simulink model "MVC3"  (R2019b)
settings: Solver=VariableStepAuto  StartTime=0.0  StopTime=SimulationTime  RelTol=1e-3
values from neighbouring files (symbols this model uses):
  disturbanceStrength = 0.001    [Obliczenia.m]
  SampleTime = 1    [Obliczenia.m]
libraries: simulink x5
settings Model: Creator=pleka  LastModifiedBy=pleka

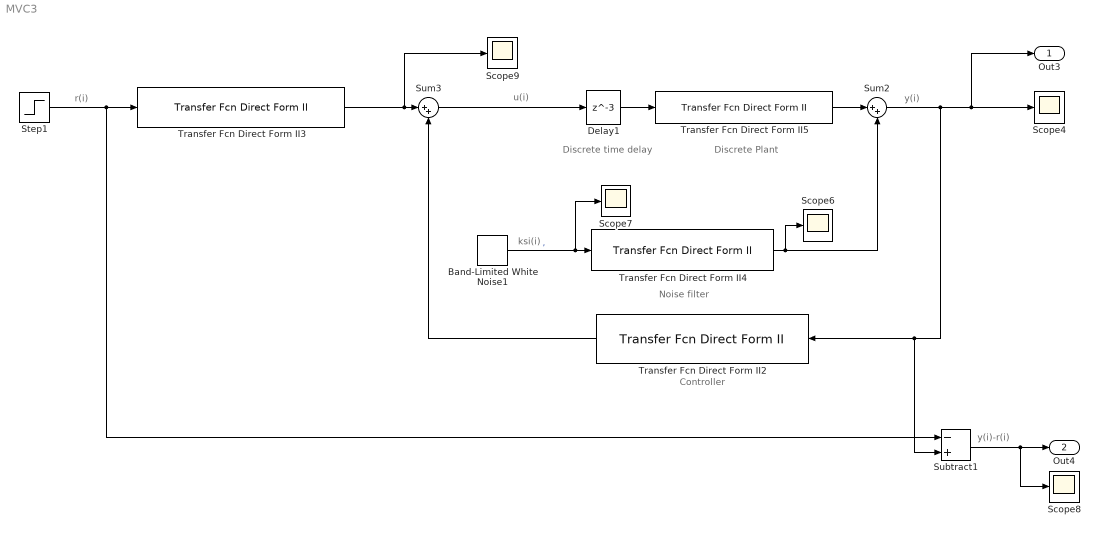
== system MVC3 ==
  note: Discrete Plant
  note: u(i)
  note: Discrete time delay
  note: Noise filter
  note: Controller
  note: r(i)
  note: y(i)-r(i)
  note: y(i)
  note: ksi(i)
  Band-Limited White Noise1 : simulink/Sources/Band-Limited White Noise  Cov=[disturbanceStrength]  Ts=SampleTime  seed=[23341]
  Delay1 : Delay  DelayLength=3
  Scope{4,6..9} (5 alike) : Scope
  Step1 : Step  After=5  SampleTime=SampleTime
  Subtract1 : Sum  Inputs=-+
  Sum2 : Sum  Inputs=|++
  Sum3 : Sum  Inputs=|++
  Transfer Fcn Direct Form II2 : simulink/Additional Math & Discrete/Additional Discrete/Transfer Fcn Direct Form II  NumCoefVec=[0.288 0.07 0 0 0]  DenCoefVec=[0.3 -0.16 0.01 0.014]  vinit=0.0  DoSatur=off
      settings: SourceProductName=Simulink  SourceProductBaseCode=SL
  Transfer Fcn Direct Form II3 : simulink/Additional Math & Discrete/Additional Discrete/Transfer Fcn Direct Form II  NumCoefVec=[1 0 0 0 0]  DenCoefVec=[0.3 -0.16 0.01 0.014]  vinit=0.0  DoSatur=off
      settings: SourceProductName=Simulink  SourceProductBaseCode=SL
  Transfer Fcn Direct Form II4 : simulink/Additional Math & Discrete/Additional Discrete/Transfer Fcn Direct Form II  NumCoefVec=[1 0 0]  DenCoefVec=[-0.8 0.5]  vinit=0.0  DoSatur=off
      settings: SourceProductName=Simulink  SourceProductBaseCode=SL
  Transfer Fcn Direct Form II5 : simulink/Additional Math & Discrete/Additional Discrete/Transfer Fcn Direct Form II  NumCoefVec=[1 -0.5 0.1]  DenCoefVec=[-0.8 0.5]  vinit=0.0  DoSatur=off
      settings: SourceProductName=Simulink  SourceProductBaseCode=SL
  Out3 : Outport
  Out4 : Outport  Port=2
  wires:
  Step1/1 -> Subtract1/1, Transfer Fcn Direct Form II3/1
  Sum3/1 -> Delay1/1
  Transfer Fcn Direct Form II4/1 -> Scope6/1, Sum2/2
  Transfer Fcn Direct Form II3/1 -> Scope9/1, Sum3/1
  Sum2/1 -> Subtract1/2, Transfer Fcn Direct Form II2/1, Out3/1, Scope4/1
  Band-Limited White Noise1/1 -> Scope7/1, Transfer Fcn Direct Form II4/1  ","
  Transfer Fcn Direct Form II2/1 -> Sum3/2
  Subtract1/1 -> Scope8/1, Out4/1
  Transfer Fcn Direct Form II5/1 -> Sum2/1
  Delay1/1 -> Transfer Fcn Direct Form II5/1
